simulink model "twolink_dynmodel_new"  (R2017a)
settings: Solver=VariableStepAuto  StartTime=0.0  StopTime=10.0  RelTol=1e-3
settings Model: Creator=Zain  LastModifiedBy=Zain

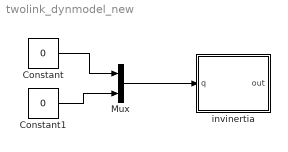
== system twolink_dynmodel_new ==
  Constant : Constant  Value=0
  Constant1 : Constant  Value=0
  Mux : Mux  Inputs=2
  invinertia : Subsystem  AncestorBlock=twolinkslib/invinertia
  wires:
  Mux/1 -> invinertia/1(q)
  Constant/1 -> Mux/1
  Constant1/1 -> Mux/2

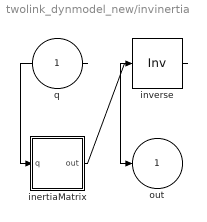
== system twolink_dynmodel_new/invinertia ==
  q : Inport
  inertiaMatrix : Subsystem  AncestorBlock=twolinkslib/inertia
  inverse : Product  Inputs=/  Multiplication=Matrix(*)
  out : Outport
  wires:
  inverse/1 -> out/1
  inertiaMatrix/1(out) -> inverse/1
  q/1 -> inertiaMatrix/1(q)

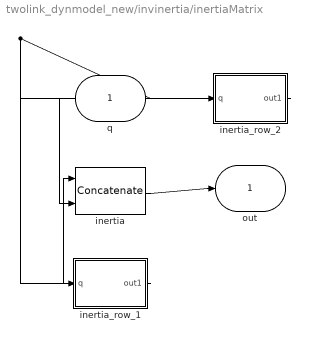
== system twolink_dynmodel_new/invinertia/inertiaMatrix ==
  q : Inport
  inertia : Concatenate  Mode=Multidimensional array
  inertia_row_1 : MATLAB Function  TreatAsAtomicUnit=on
  inertia_row_2 : MATLAB Function  TreatAsAtomicUnit=on
  out : Outport
  wires:
  inertia/1 -> out/1
  inertia_row_1/1(out1) -> inertia/1
  q/1 -> inertia_row_1/1(q), inertia_row_2/1(q)
  inertia_row_2/1(out1) -> inertia/2

== matlab function twolink_dynmodel_new/invinertia/inertiaMatrix/inertia_row_1 ==
  data: q input; out1 output
function out1 = inertia_row_1(q)
%#codegen

%    This function was generated by the Symbolic Math Toolbox version 7.2.
%    12-Mar-2019 13:59:31

q = q(:,2);
t2 = cos(q(2));
out1 = [t2+3.0./2.0,t2.*(1.0./2.0)+1.0./4.0];

== matlab function twolink_dynmodel_new/invinertia/inertiaMatrix/inertia_row_2 ==
  data: q input; out1 output
function out1 = inertia_row_2(q)
%#codegen

%    This function was generated by the Symbolic Math Toolbox version 7.2.
%    12-Mar-2019 13:59:31

q = q(:,2);
out1 = [cos(q(2)).*(1.0./2.0)+1.0./4.0,1.0./4.0];
